simulink model "ATFIDP_FlightComputer"  (R2025a)
settings: Solver=FixedStepDiscrete  StartTime=0  StopTime=60  FixedStep=0.1  RelTol=1e-3
libraries: simulink x2
settings Model: Creator=saipr  LastModifiedBy=saipr

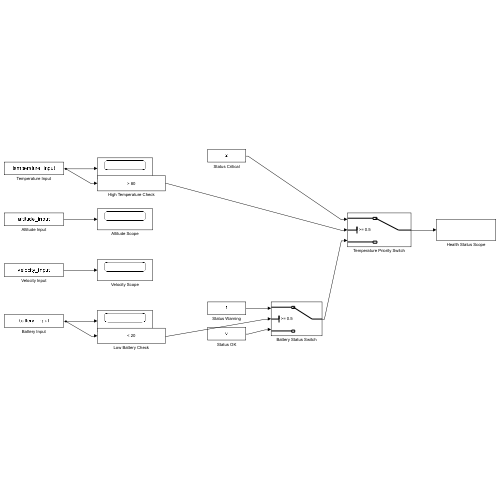
[thumbnail: Simulink's stored preview of the top-level diagram]
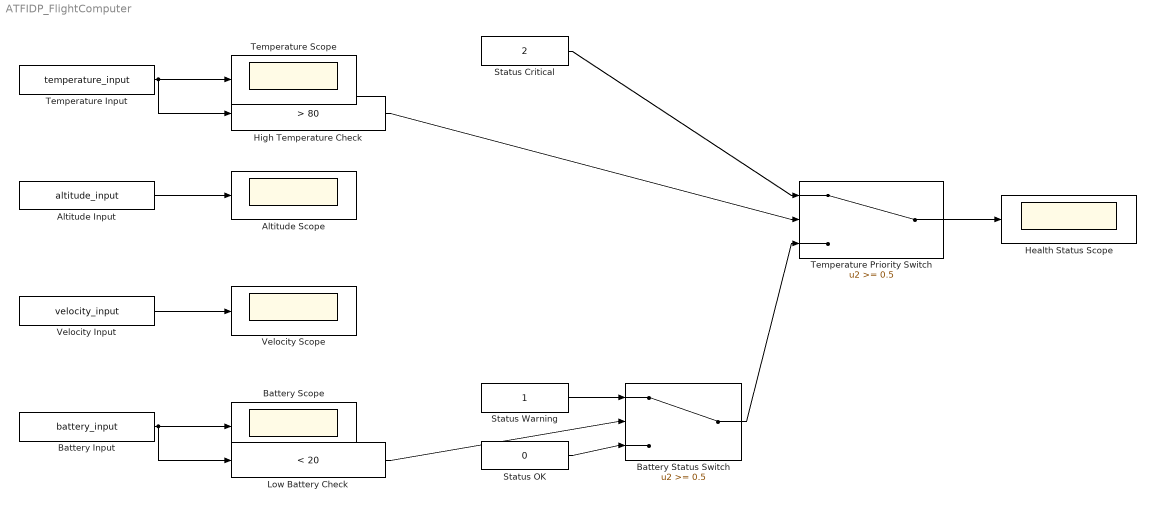
== system ATFIDP_FlightComputer ==
  Altitude Input : FromWorkspace  VariableName=altitude_input
  Altitude Scope : Scope
  Battery Input : FromWorkspace  VariableName=battery_input
  Battery Scope : Scope
  Battery Status Switch : Switch  Threshold=0.5  SaturateOnIntegerOverflow=off  InputSameDT=off
  Health Status Scope : Scope
  High Temperature Check : simulink/Logic and Bit Operations/Compare To Constant  relop=>  const=80  OutDataTypeStr=boolean
  Low Battery Check : simulink/Logic and Bit Operations/Compare To Constant  relop=<  const=20  OutDataTypeStr=boolean
  Status Critical : Constant  Value=2
  Status OK : Constant  Value=0
  Status Warning : Constant
  Temperature Input : FromWorkspace  VariableName=temperature_input
  Temperature Priority Switch : Switch  Threshold=0.5  SaturateOnIntegerOverflow=off  InputSameDT=off
  Temperature Scope : Scope
  Velocity Input : FromWorkspace  VariableName=velocity_input
  Velocity Scope : Scope
  wires:
  Temperature Input/1 -> Temperature Scope/1, High Temperature Check/1
  Altitude Input/1 -> Altitude Scope/1
  Velocity Input/1 -> Velocity Scope/1
  Battery Input/1 -> Battery Scope/1, Low Battery Check/1
  Status Warning/1 -> Battery Status Switch/1
  Status OK/1 -> Battery Status Switch/3
  Low Battery Check/1 -> Battery Status Switch/2
  Status Critical/1 -> Temperature Priority Switch/1
  Battery Status Switch/1 -> Temperature Priority Switch/3
  High Temperature Check/1 -> Temperature Priority Switch/2
  Temperature Priority Switch/1 -> Health Status Scope/1
